simulink model "Simulation_3_model"  (R2017b)
settings: Solver=FixedStepAuto  StartTime=0.0  StopTime=3  FixedStep=.0001  RelTol=1e-3
values from neighbouring files (symbols this model uses):
  Kt = 0.3    [Simulation_3_code.m]
  Tem_f = 9    [Simulation_3_code.m]
  Tem_i = 6    [Simulation_3_code.m]
  Tem_time = .3    (= 0.3)    [Simulation_3_code.m]
  Tl_f = 480    [Simulation_3_code.m]
  Tl_i = 300    [Simulation_3_code.m]
  Tl_time = 2    [Simulation_3_code.m]
libraries: powerlib x5
settings Model: Creator=Andrew McCullough  LastModifiedBy=Andrew McCullough

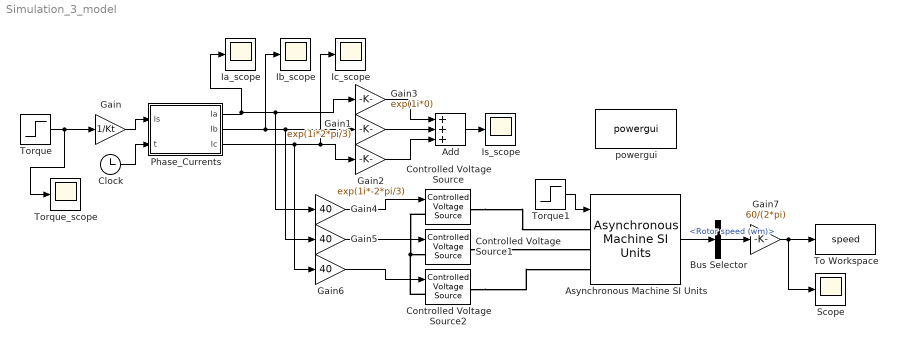
== system Simulation_3_model ==
  Add : Sum  Inputs=+++
  Asynchronous Machine SI Units : powerlib/Machines/Asynchronous Machine SI Units  RotorType=Squirrel-cage  PresetModel=No  MechanicalLoad=Torque Tm  ShowDetailedParameters=on  ReferenceFrame=Rotor  Units=SI  MeasurementBus=off  NominalParameters=[1.845e+04 400 50]  Stator=[0.5968 0.0003495]  Rotor=[0.6258 0.005473]  Cage1=[0.4155 0.002066]  Cage2=[0.4168 0.0003495]  Lm=0.0354  Mechanical=[0.05 0.005879 2]  PolePairs=2  InitialConditions=[0 0 0 0 0 0 0 0]  SimulateSaturation=off  Saturation=[14.03593122, 27.81365428, 53.79336849, 72.68890987, 97.98006896, 148.6815601, 215.7428561, 302.9841135, 428.7778367 ; 230, 322, 414, 460, 506, 552, 598, 644, 690]  LoadFlowParameters=1492000  TsPowergui=0  TsBlock=-1  IterativeModel=Trapezoidal non iterative  IterativeDiscreteModel=Trapezoidal non iterative  Pmec=1.492e+006
  Bus Selector : BusSelector  OutputSignals=Mechanical.Rotor speed (wm)
  Clock : Clock
  Controlled Voltage Source : powerlib/Electrical Sources/Controlled Voltage Source  Initialize=on  Source_Type=AC  Amplitude=0  Phase=0  Frequency=0  Measurements=None
  Controlled Voltage Source1 : powerlib/Electrical Sources/Controlled Voltage Source  Initialize=on  Source_Type=AC  Amplitude=0  Phase=0  Frequency=0  Measurements=None
  Controlled Voltage Source2 : powerlib/Electrical Sources/Controlled Voltage Source  Initialize=on  Source_Type=AC  Amplitude=0  Phase=0  Frequency=0  Measurements=None
  Gain : Gain  Gain=1/Kt
  Gain1 : Gain  Gain=exp(1i*2*pi/3)
  Gain2 : Gain  Gain=exp(1i*-2*pi/3)
  Gain3 : Gain  Gain=exp(1i*0)
  Gain4 : Gain  Gain=40
  Gain5 : Gain  Gain=40
  Gain6 : Gain  Gain=40
  Gain7 : Gain  Gain=60/(2*pi)
  Ia_scope : Scope
  Ib_scope : Scope
  Ic_scope : Scope
  Is_scope : Scope
  Phase_Currents : MATLAB Function  TreatAsAtomicUnit=on
  Scope : Scope
  To Workspace : ToWorkspace  VariableName=speed  SaveFormat=Timeseries  SampleTime=-1
  Torque : Step  Time=Tem_time  Before=Tem_i  After=Tem_f  SampleTime=0
  Torque1 : Step  Time=Tl_time  Before=Tl_i  After=Tl_f  SampleTime=0
  Torque_scope : Scope
  powergui : powerlib/powergui  Priority=1  SimulationMode=Discrete  SampleTime=.0001  frequency=60  Iterations=50  frequencyindice=50  Pbase=100e6  ErrMax=1e-4  UnitsV=kV  UnitsW=MW  buscounter=0  FunctionMessages=off  echomessages=off  EnableUseOfTLC=off  CurrentSourceSwitches=off  DisableSnubberDevices=off  DisableRonSwitches=off  DisableVfSwitches=off  DisplayEquations=off  SolverType=Tustin/Backward Euler (TBE)  Interpol=off  ExternalGateDelay=off  methode=off  Ts=100  x0status=blocks  SPID=off  SwTol=0  HookPort=off  RestoreLinks=warning  ResistiveCurrentMeasurement=off  Frange=[0:2:500]  Ylog=off  Xlog=on  ShowGrid=off  save=off  variable=ZData  structure=0  ZoomFFT=off  StartTime=0.0  cycles=1  DisplayStyle=1  fundamental=60  FreqAxis=off  MaxFrequency=1000  frequencyindicesteady=1  RmsSteady=1  display=off
  wires:
  Torque/1 -> Gain/1, Torque_scope/1
  Gain/1 -> Phase_Currents/1(Is)
  Add/1 -> Is_scope/1
  Phase_Currents/1(Ia) -> Gain4/1, Gain3/1, Ia_scope/1
  Phase_Currents/3(Ic) -> Gain6/1, Gain2/1, Ic_scope/1
  Clock/1 -> Phase_Currents/2(t)
  Gain3/1 -> Add/1
  Gain1/1 -> Add/2
  Gain2/1 -> Add/3
  Torque1/1 -> Asynchronous Machine SI Units/1
  Gain4/1 -> Controlled Voltage Source/1
  Gain5/1 -> Controlled Voltage Source1/1
  Gain6/1 -> Controlled Voltage Source2/1
  Phase_Currents/2(Ib) -> Gain5/1, Gain1/1, Ib_scope/1
  Asynchronous Machine SI Units/1 -> Bus Selector/1
  Bus Selector/1 -> Gain7/1  "<Rotor speed (wm)>"
  Gain7/1 -> To Workspace/1, Scope/1
  connections:
  Controlled Voltage Source/LConn1 -- Controlled Voltage Source2/LConn1 -- Controlled Voltage Source1/LConn1
  Controlled Voltage Source/RConn1 -- Asynchronous Machine SI Units/LConn1
  Controlled Voltage Source1/RConn1 -- Asynchronous Machine SI Units/LConn2
  Controlled Voltage Source2/RConn1 -- Asynchronous Machine SI Units/LConn3

== matlab function Simulation_3_model/Phase_Currents ==
  data: Ia output; Ib output; Is input; Ic output; t input
function [Ia, Ib, Ic]= fcn(Is,t)

w = 2*pi*60;
Is = Is*exp(1i*w*t);

Ia = (2/3)*real(Is*exp(1i*0));
Ib = (2/3)*real(Is*exp(1i*((-2*pi)/3)));
Ic = (2/3)*real(Is*exp(1i*((-4*pi)/3)));
